simulink model "lrlowpass_6"  (R2016b)
settings: Solver=ode15s  StartTime=0.0  StopTime=50  RelTol=1e-3
values from neighbouring files (symbols this model uses):
  C1 = 1e-10    [rlcsolver_total.m]
  CH = .047    (= 0.047)    [rlcsolver_total.m]
  CLw = .047    (= 0.047)    [rlcsolver_total.m]
  CtotH = 3.3e-8    (= 3.3e-08)    [rlcsolver_total.m]
  CtotL = 3.3e-8    (= 3.3e-08)    [rlcsolver_total.m]
  freq = 120    [rlcsolver_total.m]
  L1 = 100e-6    (= 0.0001)    [rlcsolver_total.m]
  LH = 1e-10    [rlcsolver_total.m]
  LLw = 1e-10    [rlcsolver_total.m]
  n1 = 0.31/12    (= 0.0258333333333)    [rlcsolver_total.m]
  n3 = 0.1/12    (= 0.00833333333333)    [rlcsolver_total.m]
  PerT = 0.025    [rlcsolver_total.m]
  PerV = 6    [rlcsolver_total.m]
  R1 = 1e-4    (= 0.0001)    [rlcsolver_total.m]
  RH = 1e-4    (= 0.0001)    [rlcsolver_total.m]
  RLw = 1e-4    (= 0.0001)    [rlcsolver_total.m]
  RtotH = .005    (= 0.005)    [rlcsolver_total.m]
  RtotL = .005    (= 0.005)    [rlcsolver_total.m]
settings Model: Creator=Brian  LastModifiedBy=Brian

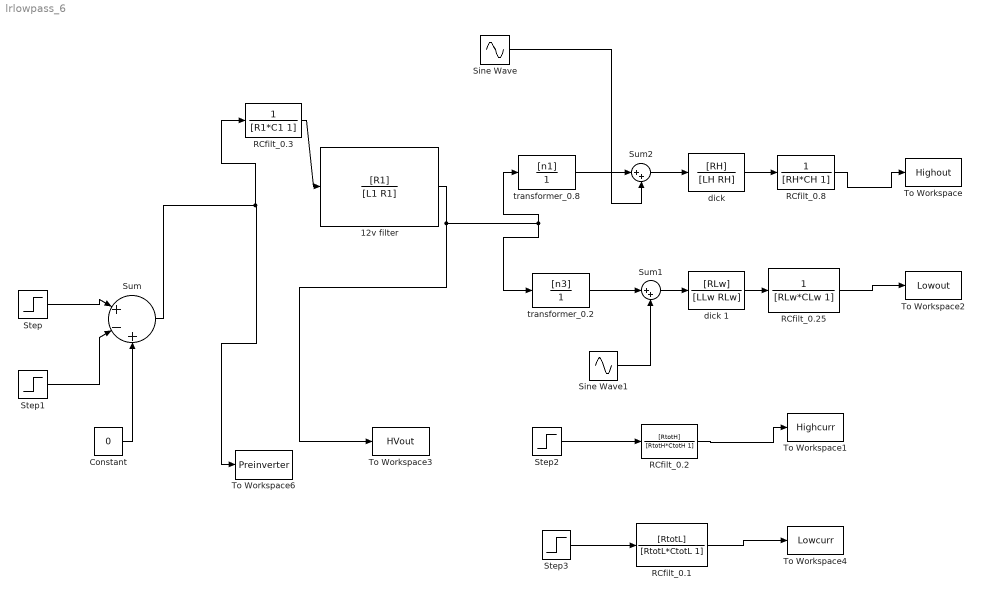
== system lrlowpass_6 ==
  12v filter : TransferFcn  Numerator=[R1]  Denominator=[L1 R1]
  Constant : Constant  Value=0
  RCfilt_0.1 : TransferFcn  Numerator=[RtotL]  Denominator=[RtotL*CtotL 1]
  RCfilt_0.2 : TransferFcn  Numerator=[RtotH]  Denominator=[RtotH*CtotH 1]
  RCfilt_0.25 : TransferFcn  Denominator=[RLw*CLw 1]
  RCfilt_0.3 : TransferFcn  Denominator=[R1*C1 1]
  RCfilt_0.8 : TransferFcn  Denominator=[RH*CH 1]
  Sine Wave : Sin  Amplitude=.002  Frequency=6.28*freq  SampleTime=0
  Sine Wave1 : Sin  Amplitude=.0002  Frequency=freq*6.28  SampleTime=0
  Step : Step  Time=0  After=PerV  SampleTime=0
  Step1 : Step  Time=PerT  After=PerV  SampleTime=0
  Step2 : Step  Time=0  After=100  SampleTime=0
  Step3 : Step  Time=0  After=100  SampleTime=0
  Sum : Sum  Inputs=|+-+
  Sum1 : Sum  Inputs=|++
  Sum2 : Sum  Inputs=|++
  To Workspace : ToWorkspace  VariableName=Highout  SaveFormat=Timeseries  SampleTime=-1
  To Workspace1 : ToWorkspace  VariableName=Highcurr  SaveFormat=Timeseries  SampleTime=-1
  To Workspace2 : ToWorkspace  VariableName=Lowout  SaveFormat=Timeseries  SampleTime=-1
  To Workspace3 : ToWorkspace  VariableName=HVout  SaveFormat=Timeseries  SampleTime=-1
  To Workspace4 : ToWorkspace  VariableName=Lowcurr  SaveFormat=Timeseries  SampleTime=-1
  To Workspace6 : ToWorkspace  VariableName=Preinverter  SaveFormat=Timeseries  SampleTime=-1
  "dick " : TransferFcn  Numerator=[RH]  Denominator=[LH RH]
  dick 1 : TransferFcn  Numerator=[RLw]  Denominator=[LLw RLw]
  transformer_0.2 : TransferFcn  Numerator=[n3]  Denominator=[1]
  transformer_0.8 : TransferFcn  Numerator=[n1]  Denominator=[1]
  wires:
  12v filter/1 -> To Workspace3/1, transformer_0.8/1, transformer_0.2/1
  Step/1 -> Sum/1
  Step1/1 -> Sum/2
  Constant/1 -> Sum/3
  RCfilt_0.8/1 -> To Workspace/1
  RCfilt_0.25/1 -> To Workspace2/1
  Sum/1 -> RCfilt_0.3/1, To Workspace6/1
  RCfilt_0.2/1 -> To Workspace1/1
  RCfilt_0.1/1 -> To Workspace4/1
  Step3/1 -> RCfilt_0.1/1
  Step2/1 -> RCfilt_0.2/1
  transformer_0.8/1 -> Sum2/1
  transformer_0.2/1 -> Sum1/1
  dick 1/1 -> RCfilt_0.25/1
  Sum1/1 -> dick 1/1
  "dick "/1 -> RCfilt_0.8/1
  Sum2/1 -> "dick "/1
  Sine Wave/1 -> Sum2/2
  Sine Wave1/1 -> Sum1/2
  RCfilt_0.3/1 -> 12v filter/1
